simulink model "sSpiegel"  (R2012b)
settings: Solver=ode45  StartTime=0.0  StopTime=10.0  RelTol=1e-3
values from neighbouring files (symbols this model uses):
  J = 93.3e-9    (= 9.33e-08)    [msSpiegel.m]    (also in msSpiegel_PID.m; msSpiegel_Pad.m; msSpiegel_Pad_Neue_Werte.m = 9.33e-09; msSpiegel_Pad_Neue_Werte_Strom.m = 9.33e-10)
  KMPHI = 6.3e-2    (= 0.063)    [msSpiegel.m]    (also in msSpiegel_PID.m; msSpiegel_Pad.m; msSpiegel_Pad_Neue_Werte.m = 0.035; msSpiegel_Pad_Neue_Werte_Strom.m = 0.035)
  LA = RA*TA    (= 0.000448)    [msSpiegel.m]    (also in msSpiegel_PID.m; msSpiegel_Pad.m; msSpiegel_Pad_Neue_Werte.m = 3e-06; msSpiegel_Pad_Neue_Werte_Strom.m = 3e-06)
  Mspiegel = 130.25e-3    (= 0.13025)    [msSpiegel.m]    (also in msSpiegel_PID.m; msSpiegel_Pad.m; msSpiegel_Pad_Neue_Werte_Strom.m = 3.025e-05)
  phi = 0.4    [Sensor_initieren.m]    (also in msSpiegel.m = 0.174532925199; msSpiegel_PID.m = 0.349065850399; msSpiegel_Pad.m = 0.349065850399; msSpiegel_Pad_Neue_Werte.m = 0.349065850399)
  r = []    [faltungsfunktionen.m]    (also in faltungsfunktionen3.m; msSpiegel.m = 6e-05; msSpiegel_PID.m = 6e-05; msSpiegel_Pad.m = 6e-05)
  RA = .16    (= 0.16)    [msSpiegel.m]    (also in msSpiegel_PID.m; msSpiegel_Pad.m; msSpiegel_Pad_Neue_Werte.m = 0.1; msSpiegel_Pad_Neue_Werte_Strom.m = 0.1)
libraries: simulink x1
settings Model: Creator=froriep  LastModifiedBy=michamann
settings DataIOCC: SignalLoggingSaveFormat=ModelDataLogs
settings DebuggingCC: FcnCallInpInsideContextMsg=EnableAllAsWarning
settings GRTTargetCC: CombineOutputUpdateFcns=off  GRTInterface=on

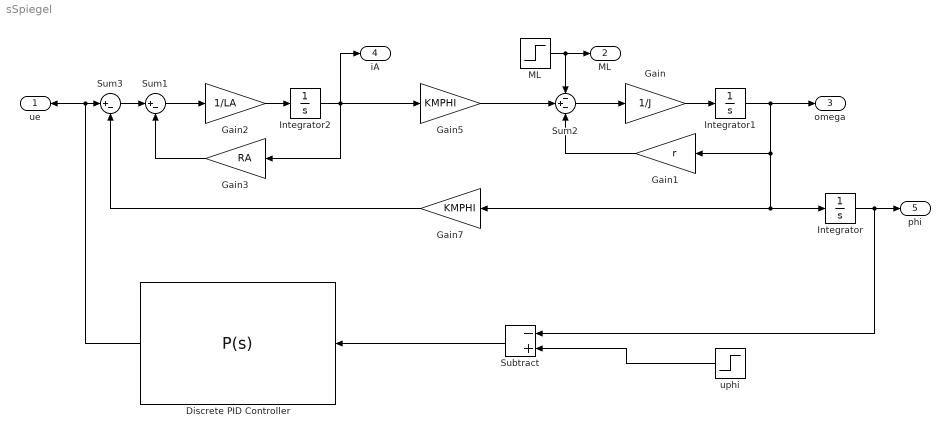
== system sSpiegel ==
  Discrete PID Controller : simulink/Continuous/PID Controller  Controller=P  TimeDomain=Continuous-time  SampleTime=1  IntegratorMethod=Trapezoidal  FilterMethod=Trapezoidal  Form=Ideal  P=800  I=0  D=0  N=0  InitialConditionSource=internal  InitialConditionForIntegrator=0  InitialConditionForFilter=0  ExternalReset=none  ZeroCross=off  LimitOutput=on  UpperSaturationLimit=24  LowerSaturationLimit=-24  LinearizeAsGain=off  AntiWindupMode=none  Kb=1  TrackingMode=off  Kt=1  RndMeth=Simplest  PParamMin=[]  PParamMax=[]  IParamMin=[]  IParamMax=[]  DParamMin=[]  DParamMax=[]  NParamMin=[]  NParamMax=[]  KbParamMin=[]  KbParamMax=[]  KtParamMin=[]  KtParamMax=[]  POutMin=[]  POutMax=[]  IOutMin=[]  IOutMax=[]  DOutMin=[]  DOutMax=[]  NOutMin=[]  NOutMax=[]  KbOutMin=[]  KbOutMax=[]  KtOutMin=[]  KtOutMax=[]  IntegratorOutMin=[]  IntegratorOutMax=[]  FilterOutMin=[]  FilterOutMax=[]  SumOutMin=[]  SumOutMax=[]  SumI1OutMin=[]  SumI1OutMax=[]  SumI2OutMin=[]  SumI2OutMax=[]  SumI3OutMin=[]  SumI3OutMax=[]  SumDOutMin=[]  SumDOutMax=[]  SaturationOutMin=[]  SaturationOutMax=[]  IntegratorContinuousStateAttributes=''  IntegratorStateMustResolveToSignalObject=off  IntegratorRTWStateStorageClass=Auto  FilterContinuousStateAttributes=''  FilterStateMustResolveToSignalObject=off  FilterRTWStateStorageClass=Auto
  Gain : Gain  Gain=1/J
  Gain1 : Gain  Gain=r
  Gain2 : Gain  Gain=1/LA
  Gain3 : Gain  Gain=RA
  Gain5 : Gain  Gain=KMPHI
  Gain7 : Gain  Gain=KMPHI
  Integrator : Integrator
  Integrator1 : Integrator
  Integrator2 : Integrator
  ML : Step  Time=0  After=Mspiegel  SampleTime=0
  Subtract : Sum  Inputs=-+
  Sum1 : Sum  Inputs=|+-
  Sum2 : Sum  Inputs=-+-
  Sum3 : Sum  Inputs=|+-
  uphi : Step  Time=100  Before=phi  After=phi  SampleTime=0
  "ue " : Outport
  "ML " : Outport  Port=2
  omega : Outport  Port=3
  iA : Outport  Port=4
  phi : Outport  Port=5
  wires:
  Integrator1/1 -> Integrator/1, Gain7/1, Gain1/1, omega/1
  Gain/1 -> Integrator1/1
  Sum2/1 -> Gain/1
  Gain1/1 -> Sum2/3
  Integrator2/1 -> Gain3/1, Gain5/1, iA/1
  Gain2/1 -> Integrator2/1
  Sum1/1 -> Gain2/1
  Gain5/1 -> Sum2/2
  ML/1 -> Sum2/1, "ML "/1
  Sum3/1 -> Sum1/1
  Gain3/1 -> Sum1/2
  Gain7/1 -> Sum3/2
  Integrator/1 -> Subtract/1, phi/1
  Discrete PID Controller/1 -> "ue "/1, Sum3/1
  Subtract/1 -> Discrete PID Controller/1
  uphi/1 -> Subtract/2
